simulink model "MultirotorSimPx4v1_8IHT"  (R2020b)
settings: Solver=VariableStepAuto  StartTime=0.0  StopTime=Simulation.T_END  MaxStep=Simulation.TS_MAX  RelTol=1e-3  EnableMultiTasking=on
PreLoadFcn:
  | % InitializeParameters;
undefined symbols (not defined in the file): Ctrl, Initial, Uav, Wind
libraries: QuaternionLibrary x14, pid_lib x7, simulink_extras x4
(part 3 of 3)

== matlab function MultirotorSimPx4v1_8IHT/Subsystem1/MATLAB Function ==
  data: q input; rates_sp output; qd input; thrust_sp input; yaw_sp_move_rate input; attitude_gain input; auto_rate_max input
function rates_sp  = control_attitude( q, qd, thrust_sp, ...
    yaw_sp_move_rate, attitude_gain, auto_rate_max )

%thrust_sp = -thrust_sp;

roll_pitch_gain = ( attitude_gain(1) + attitude_gain(2) ) / 2;
yaw_w = constrain( attitude_gain(3) / roll_pitch_gain, 0, 1 );
attitude_gain(3) = roll_pitch_gain;

q  = q  ./ norm(q);
qd = qd ./ norm(qd);

e_z   = QuatToDcmZ( q );
e_z_d = QuatToDcmZ( qd );
qd_red = VecsToQuat( e_z, e_z_d );

qd_red = QuatMult( qd_red, q );

q_mix = QuatMult( InvertQuat(qd_red), qd );
q_mix = q_mix .* SignNoZero( q_mix(1) );

q_mix(1) = constrain( q_mix(1), -1, 1 );
q_mix(4) = constrain( q_mix(4), -1, 1 );
qd = QuatMult( qd_red, ...
    [ cos( yaw_w * acos(q_mix(1)) );
    0;
    0;
    sin( yaw_w * asin(q_mix(4)) ) ] );

qe = QuatMult( InvertQuat(q), qd );

eq = 2 .* SignNoZero(qe(1)) .* qe(2:4);

rates_sp = eq .* attitude_gain;

rates_sp = rates_sp + QuatToDcmZ( InvertQuat(q) ) .* yaw_sp_move_rate;

rates_sp = constrain( rates_sp, -auto_rate_max, auto_rate_max);
end

function y = constrain( x, x_min, x_max )
    y = max( min(x, x_max), x_min );
end

function dcmZ = QuatToDcmZ( quat )
    a = quat(1);
    b = quat(2);
    c = quat(3);
    d = quat(4);
    dcmZ = [ 2 * (a * c + b * d);
        2 * (c * d - a * b);
        a * a - b * b - c * c + d * d ];
end

function quat = VecsToQuat( src, dst )
    cr = cross(src, dst);
    dt = dot(src, dst);
    quat = zeros(4,1);
    locEps = 1e-5; % Don't use eps as it's a reserved variable in MATLAB
    if (norm(cr) < locEps && dt < 0)
        % Handle corner cases with 180 degree rotations
        % If the two vectors are parallel, cross product is zero
        % If they point opposite, the dot product is negative
        cr = abs(src);
        if (cr(1) < cr(2))
            if (cr(1) < cr(3))
                cr = [1; 0; 0];
            else
                cr = [0; 0; 1];
            end
        else
            if (cr(2) < cr(3))
                cr = [0; 1; 0];
            else
                cr = [0; 0; 1];
            end
        end
        quat(1) = 0;
        cr = cross(src, cr);
    else
        % Normal case, do half-way quaternion solution
        quat(1) = dt + sqrt( norm(src)^2 * norm(dst)^2 );
    end
    quat(2) = cr(1);
    quat(3) = cr(2);
    quat(4) = cr(3);
    quat = MulticopterAttitudeControl.normalize( quat );
end

function quatInv = InvertQuat( quat )
    normSq = dot( quat, quat );
    quatInv = ( quat .* [1;-1;-1;-1] ./ normSq );
end

function quatOut = QuatMult( q1, q2 )
    quatOut = [ q1(1) * q2(1) - q1(2) * q2(2) - q1(3) * q2(3) - q1(4) * q2(4) ;
        q1(1) * q2(2) + q1(2) * q2(1) + q1(3) * q2(4) - q1(4) * q2(3) ;
        q1(1) * q2(3) - q1(2) * q2(4) + q1(3) * q2(1) + q1(4) * q2(2) ;
        q1(1) * q2(4) + q1(2) * q2(3) - q1(3) * q2(2) + q1(4) * q2(1) ];
end

function out = SignNoZero( in )
    out = ( 0 <= in ) - ( in < 0 );
end

== matlab function MultirotorSimPx4v1_8IHT/Subsystem1/MATLAB Function1 ==
  data: rate_p input; rate_i input; rate_d input; rates input; att_control output; rates_prev_filtered output; rates_sp input size=3; thrust_sp input; rates_filtered input size=3; rates_prev_filtered input size=3; rates_int output; rates_int input size=3
function [att_control, rates_prev_filtered, rates_int] = control_attitude_rates( rate_p, rate_i, rate_d, ...
    rates, rates_sp, thrust_sp, rates_filtered, rates_prev_filtered, rates_int )

    % values
    rate_int_lim = [ 0.3; 0.3; 0.3 ];
    tpa_breakpoint_p = 1;
    tpa_breakpoint_i = 1;
    tpa_breakpoint_d = 1;
    tpa_rate_p = 0;
    tpa_rate_i = 0;
    tpa_rate_d = 0;
    dt = 1/250;
    rate_ff = zeros(3,1);
    
    rates_p_scaled = rate_p .* pid_attenuations( tpa_breakpoint_p, tpa_rate_p, thrust_sp );
    rates_i_scaled = rate_i .* pid_attenuations( tpa_breakpoint_i, tpa_rate_i, thrust_sp );
    rates_d_scaled = rate_d .* pid_attenuations( tpa_breakpoint_d, tpa_rate_d, thrust_sp );

    rates_err = rates_sp - rates;

    %rates_filtered = LowPassFilter2pVector3Apply( obj, rates );

    att_control = rates_p_scaled .* rates_err + ...
        rates_int - ...
        rates_d_scaled .* (rates_filtered - rates_prev_filtered) / dt + ...
        rate_ff .* rates_sp;

    rates_prev_filtered = rates_filtered;

    rate_i_tmp = rates_int + rates_i_scaled .* rates_err .* dt;
    
    toKeep = isfinite(rate_i_tmp) & (rate_i_tmp > -rate_int_lim) & ...
                (rate_i_tmp < rate_int_lim);
    %rates_int = zeros(3,1);
    rates_int(toKeep) = rate_i_tmp(toKeep);
    
    rates_int = constrain( rates_int, -rate_int_lim, rate_int_lim );
end

function pidAttenuationPerAxis = pid_attenuations( tpa_breakpoint, tpa_rate, thrust_sp )
    TPA_RATE_LOWER_LIMIT = 0.05;
    tpa = 1.0 - tpa_rate * (abs(thrust_sp) - tpa_breakpoint) / (1.0 - tpa_breakpoint);
    tpa = max([TPA_RATE_LOWER_LIMIT, min([1.0, tpa])]);
    pidAttenuationPerAxis = [ tpa; tpa; 1.0 ];
end

function y = constrain( x, x_min, x_max )
    y = max( min(x, x_max), x_min );
end

== matlab function MultirotorSimPx4v1_8IHT/Applied wind speed/Relative velocity ==
  data: nuBody input; Uav parameter; VMotorRelBody output
function VMotorRelBody = relativeMotorVelocity( nuBody , Uav )
%#codegen
    VMotorRelBody = cross( nuBody, Uav.L_VEC );
end

== matlab function MultirotorSimPx4v1_8IHT/Applied wind speed/Compute V_app2 ==
  data: Q input; UBody output; U input size=3
function UBody = computeUBody(Q, U)
%#codegen

% Rotation matrix from Wind frame to Inertial frame
% Wind frame SEU, inertial frame NED
R_U = [1,  0, 0;
       0, -1, 0;
       0,  0, 1];
   
UBody = Q' * R_U * U;
